simulink model "EdgeDetectionVideoDM6437DVDP"  (Simulink 7.1)
settings: Solver=FixedStepDiscrete  StartTime=0.0  StopTime=10.0  RelTol=1e-3
libraries: davincilib x2, etargetslib x1, vipanalysis x1, vipconversions x1
settings Model: Creator=karin  LastModifiedBy=Administrator
settings SolverCC: PositivePriorityOrder=on
settings DataIOCC: SaveOutput=off  SaveTime=off
settings OptimizationCC: OptimizeModelRefInitCode=on
settings HardwareCC: ProdBitPerLong=40  ProdIntDivRoundTo=Zero  ProdEndianess=LittleEndian  ProdHWDeviceType=Texas Instruments->C6000
settings RTWCC: SystemTargetFile=ccslink_ert.tlc  GenCodeOnly=on  GenerateMakefile=off  TemplateMakefile=ccslink_ert.tmf  Description=Embedded IDE Link CC (ERT) code generation for TMS320(TM) DSP platforms  ProcessScript=ccslink_ert_make_rtw_hook
settings CodeAppCC: IgnoreCustomStorageClasses=off
settings ERTTgtLinkCCS: TargetFcnLib=ansi_tfl_table_tmw.mat  TargetFunctionLibrary=ANSI_C  UtilityFuncGeneration=Auto  GenerateFullHeader=on  GenerateSampleERTMain=off  GenerateTestInterfaces=off  IsPILTarget=off  ModelReferenceCompliant=on  CompOptLevelCompliant=off  IncludeMdlTerminateFcn=on  CombineOutputUpdateFcns=on  SuppressErrorStatus=off  ERTFirstTimeCompliant=off  IncludeFileDelimiter=Auto  ERTCustomFileBanners=on  SupportAbsoluteTime=on  LogVarNameModifier=rt_  MatFileLogging=off  MultiInstanceERTCode=off  SupportNonFinite=on  SupportComplex=on  PurelyIntegerCode=off  SupportContinuousTime=off  SupportNonInlinedSFcns=off  EnableShiftOperators=on  ParenthesesLevel=Nominal  PortableWordSizes=off  ModelStepFunctionPrototypeControlCompliant=off  AutosarCompliant=off  GenerateErtSFunction=off  GenerateASAP2=off  ExtMode=off  ExtModeTransport=0  ExtModeStaticAlloc=on  ExtModeStaticAllocSize=1000000  ExtModeTesting=off  ExtModeMexFile=ext_comm  ExtModeIntrfLevel=Level1  InlinedParameterPlacement=NonHierarchical  TargetOS=BareBoardExample  MultiInstanceErrorCode=Error  RateGroupingCode=on  RootIOFormat=Individual arguments  RTWCAPISignals=off  RTWCAPIParams=off  RTWCAPIStates=off  ERTSrcFileBannerTemplate=ert_code_template.cgt  ERTHdrFileBannerTemplate=ert_code_template.cgt  ERTDataSrcFileTemplate=ert_code_template.cgt  ERTDataHdrFileTemplate=ert_code_template.cgt  ERTCustomFileTemplate=example_file_process.tlc  ModuleNamingRule=Unspecified  SignalDisplayLevel=10  ParamTuneLevel=10  GlobalDataDefinition=Auto  DataDefinitionFile=global.c  GlobalDataReference=Auto  DataReferenceFile=global.h  GRTInterface=off  PreserveExpressionOrder=off  PreserveIfCondition=off  EnableUserReplacementTypes=off  MemSecPackage=--- None ---  MemSecDataConstants=Default  MemSecDataIO=Default  MemSecDataInternal=Default  MemSecDataParameters=Default  MemSecFuncInitTerm=Default  MemSecFuncExecute=Default  exportIDEObj=on  ideObjName=CCS_Obj  oldideObjName=CCS_Obj  ideObjTimeout=10  oldideObjTimeout=10  ideObjBuildTimeout=1000  oldideObjBuildTimeout=1000  ProfileGenCode=off  ProfileNumSamples=100  InlineDSPBlks=on  projectOptions=Custom  debugCompilerOptions="-g -d\"_DEBUG\""  releaseCompilerOptions=-o2  customCompilerOptions=-pm -o3  compilerOptionsStr=-pm -o3  getCompilerOptions=off  getLinkerOptions=off  systemStackSize=32768  buildAction=Build  overrunNotificationMethod=None  overrunNotificationFcn=myfunction  oldoverrunNotificationFcn=myfunction  configurePIL=off  configPILBlockAction=Create_PIL_block_build_and_download

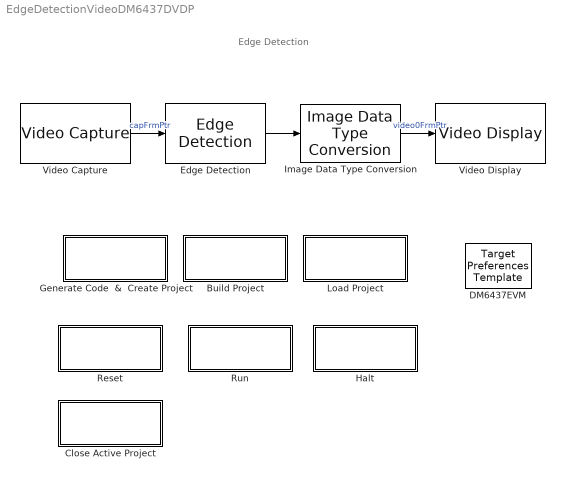
== system EdgeDetectionVideoDM6437DVDP ==
  note: Edge Detection
  Build Project : Subsystem
      settings: OpenFcn=CCS_Obj.build;
      mask Display: disp('Build\nProject')
  Close Active Project : Subsystem
      settings: OpenFcn=close(CCS_Obj,[],'project')
      mask Display: disp('Close Active Project')
  DM6437EVM : etargetslib/Target Preferences Template  Tag=ccslinktgtpref  SystemSampleTime=-1
  Edge Detection : vipanalysis/Edge Detection  DialogController=vipDDGCreate  DialogControllerArgs=DataTag1  method=Sobel  outputType=Binary image  userDefinedThreshold=off  thresholdSource=Input port  threshold=20  thresholdTuning=4  edgeThinning=off  threshold_canny=[0.25 0.60]  autoPercent=70  sigma=1  prodOutputMode=Binary point scaling  prodOutputWordLength=32  prodOutputFracLength=8  roundingMode=Floor  overflowMode=off
  Generate Code  &  Create Project : Subsystem
      settings: OpenFcn=make_rtw;
      mask Display: disp('Generate Code\n & \nCreate Project')
  Halt : Subsystem
      settings: OpenFcn=CCS_Obj.halt;
      mask Display: disp('Halt')
  Image Data Type Conversion : vipconversions/Image Data Type Conversion  outDT=uint8  isSigned=on  wordLen=16  numFracBits=0
  Load Project : Subsystem
      settings: OpenFcn=CCS_Obj.load([pwd,'\',bdroot,'_ccslink\', bdroot, '.out'])
      mask Display: disp('Load\nProject')
  Reset : Subsystem
      settings: OpenFcn=CCS_Obj.reset;
      mask Display: disp('Reset')
  Run : Subsystem
      settings: OpenFcn=CCS_Obj.run;
      mask Display: disp('Run')
  Video Capture : davincilib/Video Capture  videoCaptureMode=PAL  avInput=Composite  sampleTime=-1
  Video Display : davincilib/Video Display  videoWindow=Video0  video0Position=[0, 0, 720, 480]  video1LocSrc=Specify via dialog  video1Location=[320, 200, 152, 100]  hZoom=1x  vZoom=1x  videoEnablePort=off  videoDisplayMode=PAL  avOutput=Composite  hExpansion=off  vExpansion=off
  wires:
  Image Data Type Conversion/1 -> Video Display/1  "video0FrmPtr"
  Edge Detection/1 -> Image Data Type Conversion/1
  Video Capture/1 -> Edge Detection/1  "capFrmPtr"

== system EdgeDetectionVideoDM6437DVDP/Build Project ==

== system EdgeDetectionVideoDM6437DVDP/Close Active Project ==

== system EdgeDetectionVideoDM6437DVDP/Generate Code  &  Create Project ==

== system EdgeDetectionVideoDM6437DVDP/Halt ==

== system EdgeDetectionVideoDM6437DVDP/Load Project ==

== system EdgeDetectionVideoDM6437DVDP/Reset ==

== system EdgeDetectionVideoDM6437DVDP/Run ==
